simulink model "sampleModel1706_sub"  (R2023a)
settings: Solver=VariableStepAuto  StartTime=0.0  StopTime=10.0  RelTol=1e-3
libraries: simulink x4, hdlsllib x1
settings Model: Creator=user1  LastModifiedBy=user1
settings OptimizationCC: BlockReduction=off  ConditionallyExecuteInputs=off

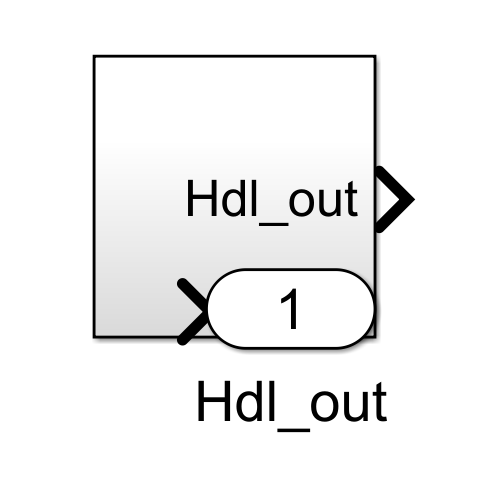
[thumbnail: Simulink's stored preview of the top-level diagram]
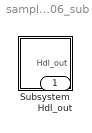
== system sampleModel1706_sub ==
  Subsystem : Subsystem
  Hdl_out : Outport  OutDataTypeStr=uint8

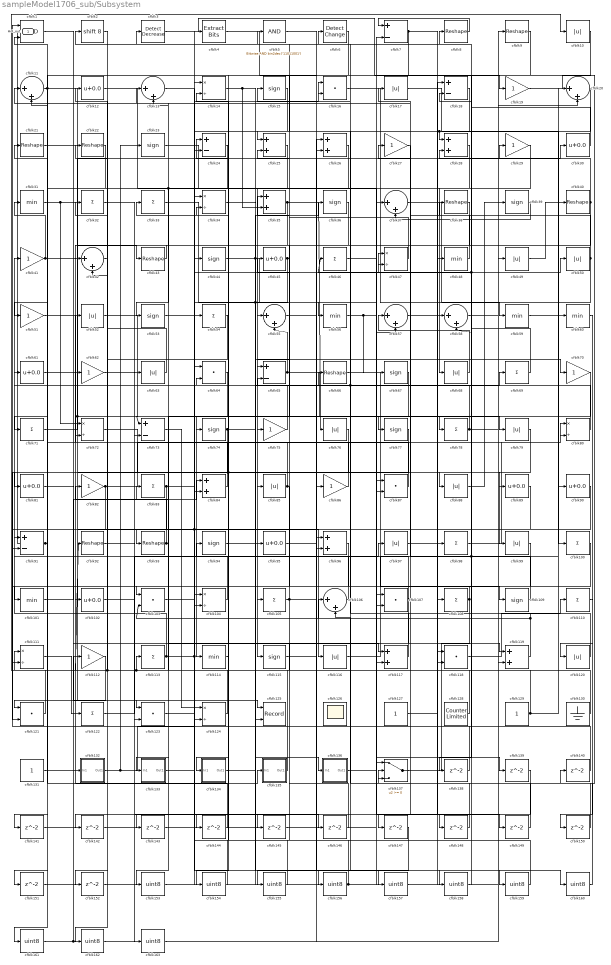
== system sampleModel1706_sub/Subsystem ==
  cfblk1 : Logic  AllPortsSameDT=off  OutDataTypeStr=boolean
  cfblk{10,17,49..50,52,63,68,76,79,85,88,97,99,116,120} (15 alike) : Abs  OutDataTypeStr=uint8  SaturateOnIntegerOverflow=off
  cfblk{32..33,46,54,69,71,78,83,98,100,105,108,110,113,122} (15 alike) : Sum  Inputs=+  OutDataTypeStr=uint8
  cfblk{31,48,56,59..60,101,114} (7 alike) : MinMax  OutDataTypeStr=uint8
  cfblk{12,30,45,61,81,89..90,95,102} (9 alike) : Bias  Bias=0.0  SaturateOnIntegerOverflow=off
  cfblk{16,64,87,103,107,118,121,123} (8 alike) : DotProduct  OutDataTypeStr=uint8
  cfblk{14,34,47,72,80,104,111,124} (8 alike) : Product  Inputs=*/  OutDataTypeStr=uint8  RndMeth=Zero  SaturateOnIntegerOverflow=on
  cfblk{11,13,20,37,42,55,57..58,106} (9 alike) : Sum  Inputs=|++  OutDataTypeStr=uint8
  cfblk{15,23,36,39,44,53,67,74,77,94,109,115} (12 alike) : Signum
  cfblk{19,27,29,41,51,62,70,75,82,86,112} (11 alike) : Gain  OutDataTypeStr=uint8
  cfblk{25..26,28,35,84,96,117,119} (8 alike) : Sum  OutDataTypeStr=uint8
  cfblk125 : Record  FileSettingsInternal="{\"entries\":[{\"content\":{\"excelSettings\":{\"content\":{},\"type\":\"Streamout.ExcelSettings\"}},\"type\":\"Streamout.FileSettingStorage\",\"uuid\":\"\"}],\"packageUris\":[\"http:\\/\\/schema.mathworks.com\\/mf0\\/streamout_blocks\\/R2020a\"],\"version\":\"1.0\"}"  Layout=[1 1]  SignalsInternal="{\"entries\":[{\"content\":{\"signals\":[{\"content\":{\"blockPath\":[],\"dimensions\":[1],\"domain\":\"\",\"lineColor\":\"#a2142f\",\"plots\":[1],\"port\":1,\"signalID\":36490,\"signalName\":\"cfblk81\"},\"type\":\"RecordBlkView.Signal\",\"uuid\":\"\"},{\"content\":{\"blockPath\":[],\"dimensions\":[1],\"domain\":\"\",\"lineColor\":\"#139fff\",\"plots\":[1],\"port\":2,\"signalID\":36493,\"signalName\":\"cfblk45\"},\"type\":\"RecordBlkView.Signal\",\"uuid\":\"\"}]},\"type\":\"RecordBlkView.InputSignals\",\"uuid\":\"\"}],\"packageUris\":[\"http:\\/\\/schema.mathworks.com\\/mf0\\/streamout_blocks\\/R2020a\"],\"version\":\"1.0\"}"  VisualizationBindings="{\"xyplotplugin\":{\"info\":[{\"series\":[{\"bindingParametersList\":[{\"parameter\":\"X-Axis\",\"signalID\":36490,\"signalName\":\"cfblk81\"},{\"parameter\":\"Y-Axis\",\"signalID\":36493,\"signalName\":\"cfblk45\"}],\"seriesID\":23689}],\"subplotID\":1}]}}"  CompatibilityTag=XY  st=-1
  cfblk126 : Scope
      settings: Floating=on
  cfblk127 : Constant  OutDataTypeStr=uint8  SampleTime=-1
  cfblk128 : hdlsllib/Sources/Counter Limited  uplimit=7  tsamp=-1
  cfblk129 : Constant  OutDataTypeStr=uint8  SampleTime=-1
  cfblk130 : Ground
  cfblk131 : Constant  OutDataTypeStr=uint8  SampleTime=-1
  cfblk132 : Subsystem
      settings: LibrarySourceBlock=|
      | hdlsllib/Ports &
      | Subsystems/Subsystem
  cfblk133 : Subsystem
      settings: LibrarySourceBlock=|
      | hdlsllib/Ports &
      | Subsystems/Subsystem
  cfblk134 : Subsystem
      settings: LibrarySourceBlock=|
      | hdlsllib/Ports &
      | Subsystems/Subsystem
  cfblk135 : Subsystem
      settings: LibrarySourceBlock=|
      | hdlsllib/Ports &
      | Subsystems/Subsystem
  cfblk136 : Subsystem
      settings: LibrarySourceBlock=|
      | hdlsllib/Ports &
      | Subsystems/Subsystem
  cfblk137 : Switch  OutDataTypeStr=uint8  SaturateOnIntegerOverflow=off  InputSameDT=off
  cfblk{138..152} (15 alike) : Delay  SampleTime=1
  cfblk{153..163} (11 alike) : DataTypeConversion  OutDataTypeStr=uint8  SaturateOnIntegerOverflow=off  RndMeth=Floor
  cfblk{7,18,24,65,73,91} (6 alike) : Sum  Inputs=+-  OutDataTypeStr=uint8
  cfblk2 : ArithShift  BitShiftNumber=8
  cfblk{8..9,21..22,38,40,43,66,92..93} (10 alike) : Reshape
  cfblk3 : simulink/Logic and Bit Operations/Detect Decrease  vinit=0.0  OutDataTypeStr=uint8
      settings: LibrarySourceBlock=|
      | hdlsllib/Logic and Bit
      | Operations/Detect
      | Decrease
  cfblk4 : simulink/Logic and Bit Operations/Extract Bits  bitsToExtract=Upper half  numBits=8  bitIdxRange=[0 7]  outScalingMode=Preserve fixed-point scaling
      settings: LibrarySourceBlock=|
      | hdlsllib/Logic and Bit
      | Operations/Extract Bits
  cfblk5 : simulink/Logic and Bit Operations/Bitwise Operator  logicop=AND  UseBitMask=on  BitMask=bin2dec('11011001')  BitMaskRealWorld=Stored Integer
      settings: LibrarySourceBlock=|
      | hdlsllib/Logic and Bit
      | Operations/Bitwise
      | Operator
  cfblk6 : simulink/Logic and Bit Operations/Detect Change  vinit=0  OutDataTypeStr=uint8
      settings: LibrarySourceBlock=|
      | hdlsllib/Logic and Bit
      | Operations/Detect
      | Change
  Hdl_out : Outport  OutDataTypeStr=uint8
  wires:
  cfblk59/1 -> cfblk60/1
  cfblk20/1 -> cfblk24/2, cfblk28/1
  cfblk28/1 -> cfblk68/1
  cfblk88/1 -> cfblk39/1
  cfblk73/1 -> cfblk124/1
  cfblk52/1 -> cfblk114/1
  cfblk67/1 -> cfblk115/1
  cfblk109/1 -> cfblk58/2, cfblk57/1
  cfblk25/1 -> cfblk85/1
  cfblk107/1 -> cfblk45/1, cfblk33/1
  cfblk98/1 -> cfblk80/1
  cfblk60/1 -> cfblk120/1
  cfblk47/1 -> cfblk2/1
  cfblk66/1 -> cfblk109/1
  cfblk8/1 -> cfblk7/1
  cfblk49/1 -> cfblk40/1
  cfblk16/1 -> cfblk108/1
  cfblk120/1 -> cfblk15/1
  cfblk22/1 -> cfblk123/1
  cfblk41/1 -> cfblk31/1, cfblk135/1(In1)
  cfblk124/1 -> cfblk22/1, cfblk92/1
  cfblk3/1 -> cfblk19/1
  cfblk35/1 -> cfblk73/2, cfblk76/1
  cfblk118/1 -> cfblk110/1
  cfblk11/1 -> cfblk71/1, cfblk88/1
  cfblk111/1 -> cfblk122/1
  cfblk122/1 -> cfblk97/1
  cfblk18/1 -> cfblk156/1
  cfblk102/1 -> cfblk123/2
  cfblk36/1 -> cfblk55/1
  cfblk50/1 -> cfblk118/2, cfblk17/1
  cfblk19/1 -> cfblk137/2
  cfblk14/1 -> cfblk35/2, cfblk77/1
  cfblk65/1 -> cfblk55/2, cfblk79/1
  cfblk12/1 -> cfblk57/2
  cfblk37/1 -> cfblk59/1
  cfblk106/1 -> cfblk41/1
  cfblk79/1 -> cfblk99/1
  cfblk17/1 -> cfblk100/1
  cfblk70/1 -> cfblk74/1
  cfblk10/1 -> cfblk25/1
  cfblk56/1 -> cfblk67/1, cfblk37/1
  cfblk129/1 -> cfblk111/1, cfblk20/1
  cfblk51/1 -> cfblk78/1
  cfblk48/1 -> cfblk11/1
  cfblk117/1 -> cfblk3/1
  cfblk33/1 -> cfblk56/1
  cfblk121/1 -> cfblk10/1
  cfblk7/1 -> cfblk89/1, cfblk51/1
  cfblk137/1 -> cfblk119/1
  cfblk61/1 -> cfblk116/1
  cfblk93/1 -> cfblk13/2, cfblk82/1
  cfblk71/1 -> cfblk73/1, cfblk30/1
  cfblk97/1 -> cfblk48/1
  cfblk90/1 -> cfblk151/1, cfblk104/2
  cfblk115/1 -> cfblk69/1
  cfblk82/1 -> cfblk111/2, cfblk80/2
  cfblk43/1 -> cfblk42/1
  cfblk105/1 -> cfblk47/2, cfblk35/1
  cfblk63/1 -> cfblk12/1
  cfblk116/1 -> cfblk90/1
  cfblk4/1 -> cfblk96/1
  cfblk113/1 -> cfblk91/1, cfblk158/1, cfblk29/1
  cfblk1/1 -> cfblk117/1
  cfblk39/1 -> cfblk37/2
  cfblk13/1 -> cfblk54/1
  cfblk40/1 -> cfblk28/2, cfblk75/1
  cfblk2/1 -> cfblk42/2
  cfblk89/1 -> cfblk102/1
  cfblk75/1 -> cfblk24/1
  cfblk23/1 -> cfblk86/1
  cfblk83/1 -> cfblk16/2, cfblk93/1
  cfblk134/1(Out1) -> cfblk136/1(In1)
  cfblk108/1 -> cfblk133/1(In1), cfblk103/1
  cfblk53/1 -> cfblk14/1
  cfblk119/1 -> cfblk103/2, cfblk38/1
  cfblk135/1(Out1) -> cfblk94/1
  cfblk68/1 -> cfblk27/1
  cfblk130/1 -> cfblk83/1
  cfblk131/1 -> cfblk112/1
  cfblk77/1 -> cfblk91/2
  cfblk100/1 -> cfblk101/1
  cfblk85/1 -> cfblk105/1, cfblk52/1
  cfblk21/1 -> cfblk43/1
  cfblk101/1 -> cfblk84/1
  cfblk132/1(Out1) -> cfblk23/1, cfblk44/1
  cfblk15/1 -> cfblk134/1(In1)
  cfblk94/1 -> cfblk36/1
  cfblk58/1 -> cfblk20/2
  cfblk32/1 -> cfblk96/2
  cfblk38/1 -> cfblk65/1
  cfblk24/1 -> cfblk141/1, cfblk53/1
  cfblk133/1(Out1) -> cfblk47/1
  cfblk112/1 -> cfblk121/1
  cfblk26/1 -> cfblk161/1
  cfblk91/1 -> Hdl_out/1, cfblk21/1
  cfblk74/1 -> cfblk66/1, cfblk81/1
  cfblk80/1 -> cfblk61/1
  cfblk87/1 -> cfblk11/2
  cfblk103/1 -> cfblk4/1
  cfblk104/1 -> cfblk13/1
  cfblk78/1 -> cfblk49/1, cfblk14/2, cfblk16/1
  cfblk99/1 -> cfblk106/2
  cfblk72/1 -> cfblk98/1
  cfblk45/1 -> cfblk25/2, cfblk125/2, cfblk124/2
  cfblk44/1 -> cfblk70/1, cfblk107/2
  cfblk127/1 -> cfblk58/1
  cfblk84/1 -> cfblk62/1
  cfblk29/1 -> cfblk84/2
  cfblk31/1 -> cfblk72/1, cfblk63/1
  cfblk55/1 -> cfblk50/1
  cfblk86/1 -> cfblk32/1
  cfblk96/1 -> cfblk121/2
  cfblk69/1 -> cfblk46/1, cfblk6/1
  cfblk81/1 -> cfblk125/1
  cfblk76/1 -> cfblk144/1, cfblk143/1
  cfblk128/1 -> cfblk72/2, cfblk113/1
  cfblk30/1 -> cfblk8/1
  cfblk114/1 -> cfblk34/2
  cfblk9/1 -> cfblk138/1
  cfblk138/1 -> cfblk1/1
  cfblk136/1(Out1) -> cfblk139/1
  cfblk140/1 -> cfblk107/1
  cfblk141/1 -> cfblk87/1
  cfblk42/1 -> cfblk142/1
  cfblk142/1 -> cfblk7/2
  cfblk143/1 -> cfblk117/2
  cfblk144/1 -> cfblk1/2
  cfblk92/1 -> cfblk145/1
  cfblk145/1 -> cfblk137/1
  cfblk123/1 -> cfblk146/1
  cfblk146/1 -> cfblk65/2
  cfblk27/1 -> cfblk147/1
  cfblk46/1 -> cfblk148/1
  cfblk148/1 -> cfblk137/3
  cfblk57/1 -> cfblk149/1
  cfblk149/1 -> cfblk106/1
  cfblk110/1 -> cfblk150/1
  cfblk150/1 -> cfblk118/1
  cfblk151/1 -> cfblk119/2
  cfblk54/1 -> cfblk152/1
  cfblk152/1 -> cfblk104/1
  cfblk64/1 -> cfblk153/1
  cfblk153/1 -> cfblk95/1
  cfblk6/1 -> cfblk154/1
  cfblk154/1 -> cfblk64/1
  cfblk147/1 -> cfblk155/1
  cfblk155/1 -> cfblk64/2
  cfblk156/1 -> cfblk34/1, cfblk87/2
  cfblk95/1 -> cfblk157/1
  cfblk157/1 -> cfblk18/1
  cfblk158/1 -> cfblk18/2
  cfblk34/1 -> cfblk159/1
  cfblk159/1 -> cfblk5/1
  cfblk5/1 -> cfblk160/1
  cfblk160/1 -> cfblk140/1
  cfblk161/1 -> cfblk9/1, cfblk132/1(In1)
  cfblk139/1 -> cfblk162/1
  cfblk162/1 -> cfblk26/1
  cfblk62/1 -> cfblk163/1
  cfblk163/1 -> cfblk26/2

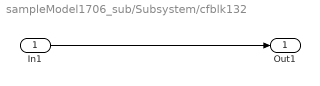
== system sampleModel1706_sub/Subsystem/cfblk132 ==
  In1 : Inport
  Out1 : Outport
  wires:
  In1/1 -> Out1/1

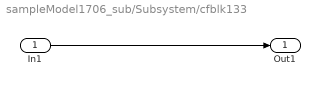
== system sampleModel1706_sub/Subsystem/cfblk133 ==
  In1 : Inport
  Out1 : Outport
  wires:
  In1/1 -> Out1/1

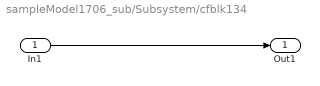
== system sampleModel1706_sub/Subsystem/cfblk134 ==
  In1 : Inport
  Out1 : Outport
  wires:
  In1/1 -> Out1/1

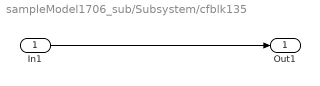
== system sampleModel1706_sub/Subsystem/cfblk135 ==
  In1 : Inport
  Out1 : Outport
  wires:
  In1/1 -> Out1/1

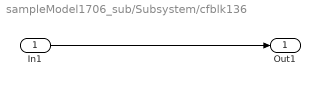
== system sampleModel1706_sub/Subsystem/cfblk136 ==
  In1 : Inport
  Out1 : Outport
  wires:
  In1/1 -> Out1/1
